simulink model "NeuromuscularModel2"  (R2019b)
settings: Solver=ode15s  StartTime=0.0  StopTime=20  MaxStep=.01  RelTol=1e-4  AbsTol=1e-6  EnableMultiTasking=on
values from neighbouring files (symbols this model uses):
  LceOffsetTA = 1-0.5*w    [ControlParams2.m]
  legLengthClr = .9    (= 0.9)    [ControlParams2.m]    (also in assignGains.m = Gains(20); assignGains2.m = Gains(20); assignGainsSagittal.m = GainsSagittal(39))
  LongDelay = 0.020    (= 0.02)    [ControlParams2.m]
  MidDelay = 0.010    (= 0.01)    [ControlParams2.m]
  N = 82    [vcmaes_1.5cm_0.9ms_Umb10_kneelim1_mstoptorque2.mat]
  ShortDelay = 0.005    [ControlParams2.m]
  simbiconGainD = 5*pi/180    (= 0.0872664625997)    [ControlParams2.m]    (also in assignGains.m = Gains(21); assignGains2.m = Gains(21); assignGainsSagittal.m = GainsSagittal(41))
  simbiconGainV = 5*pi/180    (= 0.0872664625997)    [ControlParams2.m]    (also in assignGains.m = Gains(22); assignGains2.m = Gains(22); assignGainsSagittal.m = GainsSagittal(42))
  simbiconLegAngle0 = 85*pi/180    (= 1.4835298642)    [ControlParams2.m]    (also in assignGains.m = Gains(23); assignGains2.m = Gains(23); assignGainsSagittal.m = GainsSagittal(40))
undefined symbols (not defined in the file or in its folder): footCenterToCGDist, footInertia, footMass, g, loptGAS, loptTA, lslackGAS, phimaxGASa, phimaxGASk, phirefGASa, phirefGASk, rGASa, rGASk, rhoGASa, rhoGASk, X, Y, Z
libraries: NeuroMuscularLibrary x89, nesl_utility x29, sm_lib x23, simulink x4, simulink_extras x2
(part 1 of 3)
settings Model: SimulationMode=rapid-accelerator  ParamWorkspaceSource=ReferencedWorkspace  ExtModeTrigDuration=100  TunableVars=GainGAS,GainGLU,GainHAM,GainKneeOverExt,GainSOL,GainSOLTA,GainTA,GainVAS,Kglu,PosGainGG,SpeedGainGG,groundTheta,groundX,groundZ,hipDGain,hipPGain,kneeExtendGain,kneeFlexGain,kneeHoldGain1,kneeHoldGain2,kneeStopGain,legAngleFilter,legLengthClr,simbiconGainD,simbiconGainV,simbiconLegAngle0  TunableVarsStorageClass=Auto,Auto,Auto,Auto,Auto,Auto,Auto,Auto,Auto,Auto,Auto,Auto,Auto,Auto,Auto,Auto,Auto,Auto,Auto,Auto,Auto,Auto,Auto,Auto,Auto,Auto  TunableVarsTypeQualifier=,,,,,,,,,,,,,,,,,,,,,,,,,  Creator=nitisht  LastModifiedBy=Nathan
settings SolverCC: AutoScaleAbsTol=off  ZeroCrossAlgorithm=Adaptive
settings DataIOCC: LimitDataPoints=on  SaveFinalState=on  SaveFormat=StructureWithTime  SaveOutput=off  SaveState=on  ReturnWorkspaceOutputs=off  StateSaveName=tmp_raccel_xout  SignalLoggingName=tmp_raccel_logsout
settings OptimizationCC: DefaultParameterBehavior=Inlined  EfficientMapNaN2IntZero=off  LifeSpan=inf  SimCompilerOptimization=on  AccelVerboseBuild=on
settings DebuggingCC: SaveWithDisabledLinksMsg=none  UnderspecifiedInitializationDetection=Classic  MergeDetectMultiDrivingBlocksExec=none  IgnoredZcDiagnostic=none  SolverPrmCheckMsg=warning  StateNameClashWarn=warning  SFUnexpectedBacktrackingDiag=warning  SFNoUnconditionalDefaultTransitionDiag=warning  SFExecutionAtInitializationDiag=none  ArithmeticOperatorsInVariantConditions=warning
settings HardwareCC: ProdBitPerPointer=32  ProdBitPerSizeT=32  ProdBitPerPtrDiffT=32  ProdLargestAtomicFloat=None  ProdIntDivRoundTo=Undefined  ProdEndianess=Unspecified  ProdWordSize=32  ProdHWDeviceType=Generic->Unspecified (assume 32-bit Generic)  TargetBitPerPointer=64  TargetBitPerSizeT=64  TargetBitPerPtrDiffT=64  TargetLongLongMode=on  TargetIntDivRoundTo=Zero  TargetEndianess=LittleEndian  TargetWordSize=64  TargetHWDeviceType=MATLAB Host  ProdEqTarget=off
settings ModelReferenceCC: PropagateSignalLabelsOutOfModel=off
settings SFSimCC: SFSimEcho=off  SimUseLocalCustomCode=off  CustomCodeUndefinedFunction=UseInterfaceOnly
settings RTWCC: SystemTargetFile=raccel.tlc  TemplateMakefile=raccel_default_tmf  RTWUseLocalCustomCode=off  RTWUseSimCustomCode=on
settings CodeAppCC: GenerateComments=off  MaxIdLength=128  MangleLength=10  SimulinkBlockComments=off
settings RaccelTargetCC: GeneratePreprocessorConditionals=Disable all  MultiInstanceERTCode=off  PreserveStateflowLocalDataDimensions=off  ENABLE_SLEXEC_SSBRIDGE=0  RTWCAPIParams=off
settings ConfigComp: CovMetricSettings=dw  CovHtmlReporting=on  CovSaveCumulativeToWorkspaceVar=on  CovSaveSingleToWorkspaceVar=on  CovExternalEMLEnable=off  CovSFcnEnable=off
settings SimscapeCC: SimscapeNormalizeSystem=off
settings ConfigurationSet: Description=SimMechanics 2G

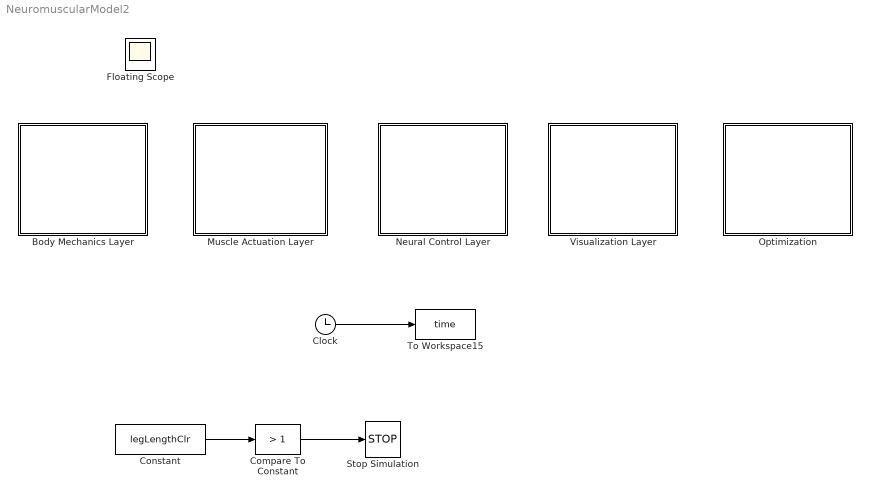
== system NeuromuscularModel2 ==
  Body Mechanics Layer : Subsystem
  Clock : Clock
  Compare To Constant : simulink/Logic and Bit Operations/Compare To Constant  relop=>  const=1  OutDataTypeStr=boolean
  Constant : Constant  Value=legLengthClr
  Muscle Actuation Layer : Subsystem
  Neural Control Layer : Subsystem
  Optimization : Subsystem
  Stop Simulation : Stop
  To Workspace15 : ToWorkspace  VariableName=time  SampleTime=-1
      settings: MaxDataPoints=1
  Visualization Layer : Subsystem
  Floating Scope : Scope
  wires:
  Clock/1 -> To Workspace15/1
  Compare To Constant/1 -> Stop Simulation/1
  Constant/1 -> Compare To Constant/1
